simulink model "zad3_model"  (R2018a)
settings: Solver=VariableStepAuto  StartTime=0.0  StopTime=1000  RelTol=1e-3
libraries: dspsrcs4 x1
settings Model: Creator=johnb  LastModifiedBy=johnb

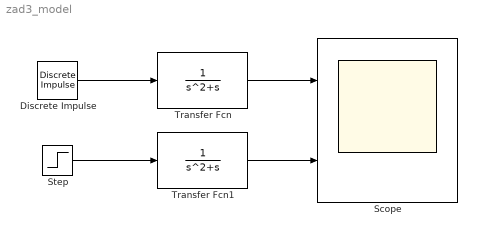
== system zad3_model ==
  Discrete Impulse : dspsrcs4/Discrete  Impulse  Delay=0  SampleTime=1  FrameSample=1  OutputFrames=off  dataType=double  isSigned=on  wordLen=16  udDataType=sfix(16)  fracBitsMode=Best precision  numFracBits=15  OutDataTypeStr=double  LastOutDataTypeStr=double
  Scope : Scope  NumInputPorts=2
  Step : Step  SampleTime=0
  Transfer Fcn : TransferFcn  Denominator=[1 1 0]
  Transfer Fcn1 : TransferFcn  Denominator=[1 1 0]
  wires:
  Discrete Impulse/1 -> Transfer Fcn/1
  Step/1 -> Transfer Fcn1/1
  Transfer Fcn1/1 -> Scope/2
  Transfer Fcn/1 -> Scope/1
